simulink model "kamman_fers"  (R2024b)
settings: Solver=VariableStepAuto  StartTime=0.0  StopTime=1000.0  RelTol=1e-3
undefined symbols (not defined in the file or in its folder): Continuous, Time
libraries: ctrlSharedLib x1
settings Model: Creator=klyx  LastModifiedBy=klyx

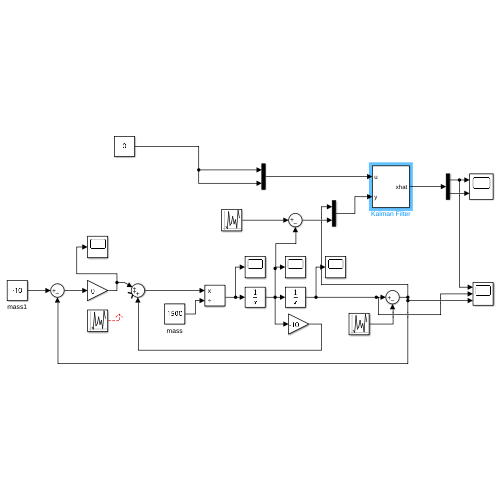
[thumbnail: Simulink's stored preview of the top-level diagram]
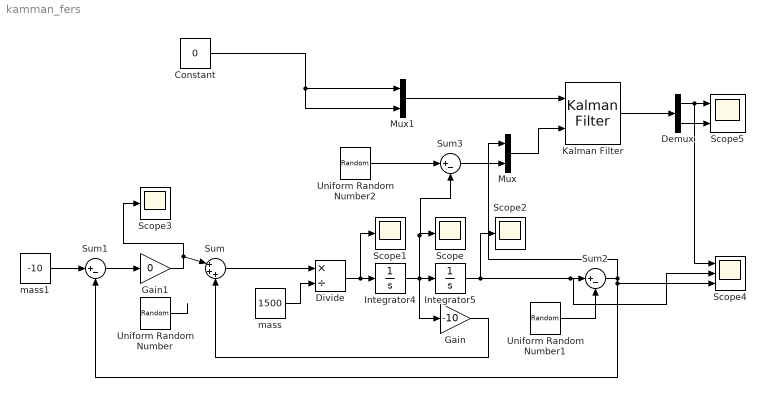
== system kamman_fers ==
  Constant : Constant  Value=0
  Demux : Demux  Outputs=2
  Divide : Product  Inputs=*/
  Gain : Gain  Gain=-10
  Gain1 : Gain  Gain=0
  Integrator4 : Integrator  InitialCondition=0.5
  Integrator5 : Integrator
  Kalman Filter : ctrlSharedLib/Kalman Filter  TimeDomain=Continuous-Time  UseCurrentEstimator=on  ModelSource=Individual A, B, C, D matrices  ModelSourceVariable=ss(0.95,1,1,0,1)  A=[0,1;0,-10/1500]  B=[0,0;0,1]  C=[1,0;0,1]  D=0  NumberOfStates=1  NumberOfInputs=1  NumberOfOutputs=1  InitialEstimateSource=Dialog  X0=0  P0=10  UseK=off  UseGH=off  NumberOfProcessNoiseInputs=1  G=1  TimeInvariantG=on  H=0  TimeInvariantH=on  Q=0.05  TimeInvariantQ=on  R=1  TimeInvariantR=on  N=0  TimeInvariantN=on  AddInputPort=on  AddEnablePort=off  OutputEstimatedY=off  OutputP=off  Ts=-1
  Mux : Mux  Inputs=2
  Mux1 : Mux  Inputs=2
  Scope{,1..3} (4 alike) : Scope
  Scope4 : Scope  NumInputPorts=3
  Scope5 : Scope  NumInputPorts=2
  Sum : Sum  Inputs=|+++
  Sum1 : Sum  Inputs=|+-
  Sum2 : Sum  Inputs=|+-
  Sum3 : Sum  Inputs=|+-
  Uniform Random Number : UniformRandomNumber  Seed=1  SampleTime=1
  Uniform Random Number1 : UniformRandomNumber  Minimum=-2  Maximum=2  Seed=1  SampleTime=1
  Uniform Random Number2 : UniformRandomNumber  Seed=1  SampleTime=1
  mass : Constant  Value=1500
  mass1 : Constant  Value=-10
  wires:
  Divide/1 -> Scope1/1, Integrator4/1
  Integrator4/1 -> Sum3/2, Scope/1, Gain/1, Integrator5/1
  Sum/1 -> Divide/1
  mass/1 -> Divide/2
  Gain/1 -> Sum/3
  Integrator5/1 -> Scope4/2, Sum2/1, Scope2/1
  Gain1/1 -> Scope3/1, Sum/1
  Sum1/1 -> Gain1/1
  mass1/1 -> Sum1/1
  Uniform Random Number/1 -> ?
  Uniform Random Number1/1 -> Sum2/2
  Sum2/1 -> Sum1/2, Scope4/3, Mux/1
  Mux/1 -> Kalman Filter/2
  Mux1/1 -> Kalman Filter/1
  Constant/1 -> Mux1/2, Mux1/1
  Kalman Filter/1 -> Demux/1
  Demux/1 -> Scope4/1, Scope5/1
  Demux/2 -> Scope5/2
  Uniform Random Number2/1 -> Sum3/1
  Sum3/1 -> Mux/2
